simulink model "DCmotor"  (R2020a)
settings: Solver=VariableStepAuto  StartTime=0.0  StopTime=3  RelTol=1e-3
model workspace (MAT data in the model file):
  SDO_OutputTimes = [0; 0.1; 0.2; 0.3; 0.4; 0.5; 0.6; 0.7; 0.8; 0.9; 1; 1.1; 1.2; 1.3; 1.4; 1.5; 1.6; 1.7; 1.8; 1.9; 2; 2.1; 2.2; 2.3; 2.4; 2.5; 2.6; 2.7; 2.8; 2.9; 3]
values from neighbouring files (symbols this model uses):
  b = 0.1    [DCmotormat.m]    (also in rough.m = [0 K])
  J = 0.01    [DCmotormat.m]    (also in rough.m = 1)
  Kb = 0.01    [DCmotormat.m]
  Kt = 0.01    [DCmotormat.m]
  L = 0.5    [DCmotormat.m]
  R = 1    [DCmotormat.m]
settings Model: OrderedModelArguments=off  Creator=hp  LastModifiedBy=hp
settings DataIOCC: OutputOption=AdditionalOutputTimes  OutputTimes=SDO_OutputTimes  ReturnWorkspaceOutputsName=SDOSimTest_Log

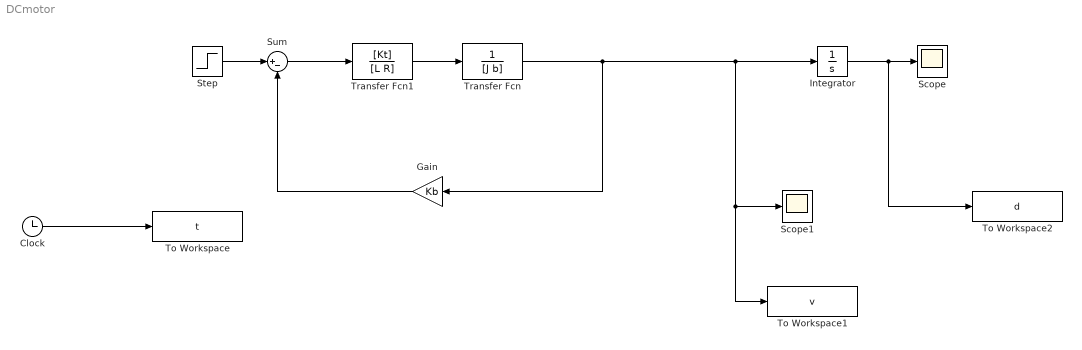
== system DCmotor ==
  Clock : Clock
  Gain : Gain  Gain=Kb
  Integrator : Integrator
  Scope : Scope
  Scope1 : Scope
  Step : Step  Time=0  After=6  SampleTime=0
  Sum : Sum  Inputs=|+-
  To Workspace : ToWorkspace  VariableName=t  SampleTime=-1
  To Workspace1 : ToWorkspace  VariableName=v  SampleTime=-1
  To Workspace2 : ToWorkspace  VariableName=d  SampleTime=-1
  Transfer Fcn : TransferFcn  Denominator=[J b]
  Transfer Fcn1 : TransferFcn  Numerator=[Kt]  Denominator=[L R]
  wires:
  Step/1 -> Sum/1
  Transfer Fcn/1 -> Gain/1, To Workspace1/1, Scope1/1, Integrator/1
  Transfer Fcn1/1 -> Transfer Fcn/1
  Gain/1 -> Sum/2
  Integrator/1 -> To Workspace2/1, Scope/1
  Sum/1 -> Transfer Fcn1/1
  Clock/1 -> To Workspace/1
